simulink library "constThr_cl"  (R2020a)
settings: Solver=VariableStepAuto  StartTime=0.0  StopTime=10.0  RelTol=1e-3
undefined symbols (not defined in the file): wnch
settings Model: Creator=mcobb  LastModifiedBy=andre
settings DataIOCC: ReturnWorkspaceOutputs=off
settings DebuggingCC: ArithmeticOperatorsInVariantConditions=warning
settings SFSimCC: CustomCodeUndefinedFunction=UseInterfaceOnly

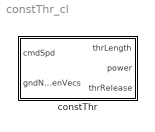
== system constThr_cl ==
  constThr : Subsystem  VariantControl=VSS_winch_winch000

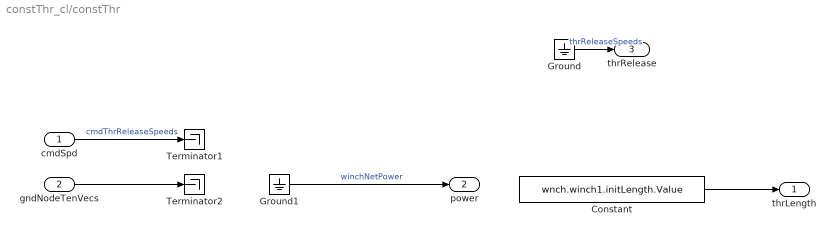
== system constThr_cl/constThr ==
  cmdSpd : Inport
  gndNodeTenVecs : Inport  Port=2
  Constant : Constant  Value=wnch.winch1.initLength.Value  VectorParams1D=off
  Ground : Ground
  Ground1 : Ground
  Terminator1 : Terminator
  Terminator2 : Terminator
  thrLength : Outport  VectorParamsAs1DForOutWhenUnconnected=off
  power : Outport  Port=2  VectorParamsAs1DForOutWhenUnconnected=off
  "thrRelease " : Outport  Port=3  VectorParamsAs1DForOutWhenUnconnected=off
  wires:
  gndNodeTenVecs/1 -> Terminator2/1
  Ground/1 -> "thrRelease "/1  "thrReleaseSpeeds"
  Ground1/1 -> power/1  "winchNetPower"
  Constant/1 -> thrLength/1
  cmdSpd/1 -> Terminator1/1  "cmdThrReleaseSpeeds"
